simulink model "sistema_omega"  (Simulink 8.4)
settings: Solver=ode4  SolverMode=SingleTasking  StartTime=0.0  StopTime=tfin+ts  FixedStep=ts  MaxStep=ts  RelTol=1e-6  AbsTol=1e-9
undefined symbols (not defined in the file): alfa1, th, ts
settings Model: Creator=zamora  LastModifiedBy=zamora  ExtModeTrigMode=oneshot  ExtModeArmWhenConnect=off  BufferReuse=off
settings SolverCC: ZeroCrossAlgorithm=Adaptive
settings DataIOCC: LimitDataPoints=off  SaveOutput=off  SaveTime=off  StateSaveName=x  TimeSaveName=t  OutputSaveName=y
settings OptimizationCC: BlockReduction=off  BooleanDataType=off  InlineParams=on  BufferReuse=off
settings DebuggingCC: SaveWithParameterizedLinksMsg=none  SignalResolutionControl=TryResolveAllWithWarning  MaxConsecutiveZCsMsg=none  IgnoredZcDiagnostic=none  SolverPrmCheckMsg=none  MultiTaskDSMMsg=warning  MultiTaskCondExecSysMsg=none  FcnCallInpInsideContextMsg=EnableAllAsWarning
settings HardwareCC: TargetUnknown=on
settings RTWCC: TemplateMakefile=grt_unix.tmf  IncludeERTFirstTime=on

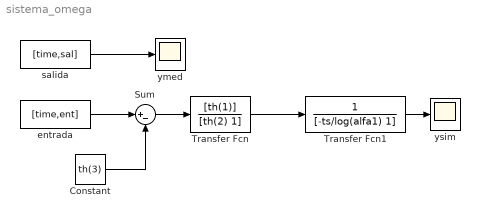
== system sistema_omega ==
  Constant : Constant  Value=th(3)  SampleTime=0
  Sum : Sum  Inputs=|+-
  Transfer Fcn : TransferFcn  Numerator=[th(1)]  Denominator=[th(2) 1]
  Transfer Fcn1 : TransferFcn  Numerator=1  Denominator=[-ts/log(alfa1) 1]
  entrada : FromWorkspace  VariableName=[time,ent]  SampleTime=ts
  salida : FromWorkspace  VariableName=[time,sal]  SampleTime=ts
  ymed : Scope
      settings: SaveName=ymed  SampleInput=on  SampleTime=ts
  ysim : Scope
      settings: SaveName=ysim  SampleInput=on  SampleTime=ts
  wires:
  salida/1 -> ymed/1
  Transfer Fcn1/1 -> ysim/1
  Transfer Fcn/1 -> Transfer Fcn1/1
  entrada/1 -> Sum/1
  Sum/1 -> Transfer Fcn/1
  Constant/1 -> Sum/2
